simulink model "case7"  (R2024b)
settings: Solver=FixedStepAuto  StartTime=0  StopTime=1  FixedStep=1e-7  RelTol=1e-3
values from neighbouring files (symbols this model uses):
  SG_D_1_D = 0.01056    [IEEE9_case_parameters.m]    (also in case1_parameters.m; case2_parameters.m; case3_parameters.m; case4_parameters.m)
  SG_D_1_EnableSaturation = 0    [IEEE9_case_parameters.m]    (also in case1_parameters.m; case2_parameters.m; case3_parameters.m; case4_parameters.m)
  SG_D_1_f0 = 60    [IEEE9_case_parameters.m]    (also in case1_parameters.m; case2_parameters.m; case3_parameters.m; case4_parameters.m)
  SG_D_1_H = 7.5    [IEEE9_case_parameters.m]    (also in case1_parameters.m; case2_parameters.m; case3_parameters.m; case4_parameters.m)
  SG_D_1_K_A = 20    [IEEE9_case_parameters.m]    (also in case1_parameters.m; case2_parameters.m; case3_parameters.m; case4_parameters.m)
  SG_D_1_K_E = 1.000000e+1    (= 10)    [IEEE9_case_parameters.m]    (also in case1_parameters.m; case2_parameters.m; case3_parameters.m; case4_parameters.m)
  SG_D_1_K_F = 2.363    [IEEE9_case_parameters.m]    (also in case1_parameters.m; case2_parameters.m; case3_parameters.m; case4_parameters.m)
  SG_D_1_K_s = 0.5    [IEEE9_case_parameters.m]    (also in case1_parameters.m = 5; case2_parameters.m = 5; case3_parameters.m = 5; case4_parameters.m = 5)
  SG_D_1_R_a = 0.001088    [IEEE9_case_parameters.m]    (also in case1_parameters.m; case2_parameters.m; case3_parameters.m; case4_parameters.m)
  SG_D_1_S_A = 1    [IEEE9_case_parameters.m]    (also in case1_parameters.m; case2_parameters.m; case3_parameters.m; case4_parameters.m)
  SG_D_1_S_B = 0.103    [IEEE9_case_parameters.m]    (also in case1_parameters.m; case2_parameters.m; case3_parameters.m; case4_parameters.m)
  SG_D_1_S_N = 10.659857    [IEEE9_case_parameters.m]    (also in case1_parameters.m; case2_parameters.m; case3_parameters.m; case4_parameters.m)
  SG_D_1_SpeedPara = 200    [IEEE9_case_parameters.m]    (also in case1_parameters.m; case2_parameters.m; case3_parameters.m; case4_parameters.m)
  SG_D_1_T_0 = 0.720173    [IEEE9_case_parameters.m]    (also in case1_parameters.m = 0.755522; case2_parameters.m = 0.808931; case3_parameters.m = 0.869402; case4_parameters.m = 0.729316)
  SG_D_1_T_1 = 0.3    [IEEE9_case_parameters.m]    (also in case1_parameters.m; case2_parameters.m; case3_parameters.m; case4_parameters.m)
  SG_D_1_T_2 = 0.05    [IEEE9_case_parameters.m]    (also in case1_parameters.m; case2_parameters.m; case3_parameters.m; case4_parameters.m)
  SG_D_1_T_3 = 0.02    [IEEE9_case_parameters.m]    (also in case1_parameters.m; case2_parameters.m; case3_parameters.m; case4_parameters.m)
  SG_D_1_T_4 = 0.005    [IEEE9_case_parameters.m]    (also in case1_parameters.m; case2_parameters.m; case3_parameters.m; case4_parameters.m)
  SG_D_1_T_A = 0.02    [IEEE9_case_parameters.m]    (also in case1_parameters.m; case2_parameters.m; case3_parameters.m; case4_parameters.m)
  SG_D_1_T_dd = 8.000000e+0    (= 8)    [IEEE9_case_parameters.m]    (also in case1_parameters.m; case2_parameters.m; case3_parameters.m; case4_parameters.m)
  SG_D_1_T_ddd = 0.04    [IEEE9_case_parameters.m]    (also in case1_parameters.m; case2_parameters.m; case3_parameters.m; case4_parameters.m)
  SG_D_1_T_E = 0.314    [IEEE9_case_parameters.m]    (also in case1_parameters.m; case2_parameters.m; case3_parameters.m; case4_parameters.m)
  SG_D_1_T_F = 0.35    [IEEE9_case_parameters.m]    (also in case1_parameters.m; case2_parameters.m; case3_parameters.m; case4_parameters.m)
  SG_D_1_T_qd = 0.8    [IEEE9_case_parameters.m]    (also in case1_parameters.m; case2_parameters.m; case3_parameters.m; case4_parameters.m)
  SG_D_1_T_qdd = 0.02    [IEEE9_case_parameters.m]    (also in case1_parameters.m; case2_parameters.m; case3_parameters.m; case4_parameters.m)
  SG_D_1_T_speed = 0.1    [IEEE9_case_parameters.m]    (also in case1_parameters.m = 200; case2_parameters.m = 200; case3_parameters.m = 200; case4_parameters.m = 200)
  SG_D_1_T_w = 0.5    [IEEE9_case_parameters.m]    (also in case1_parameters.m; case2_parameters.m; case3_parameters.m; case4_parameters.m)
  SG_D_1_V_ref = 1.990276    [IEEE9_case_parameters.m]    (also in case1_parameters.m = 2.042296; case2_parameters.m = 2.051388; case3_parameters.m = 2.089584; case4_parameters.m = 2.01845)
  SG_D_1_w_ref = 376.991118    [IEEE9_case_parameters.m]    (also in case1_parameters.m; case2_parameters.m; case3_parameters.m; case4_parameters.m)
  SG_D_1_wb = 6.000000e+1    (= 60)    [IEEE9_case_parameters.m]    (also in case1_parameters.m; case2_parameters.m; case3_parameters.m; case4_parameters.m)
  SG_D_1_x_d = 1.9    [IEEE9_case_parameters.m]    (also in case1_parameters.m; case2_parameters.m; case3_parameters.m; case4_parameters.m)
  SG_D_1_x_dd = 0.302    [IEEE9_case_parameters.m]    (also in case1_parameters.m; case2_parameters.m; case3_parameters.m; case4_parameters.m)
  SG_D_1_x_ddd = 0.204    [IEEE9_case_parameters.m]    (also in case1_parameters.m; case2_parameters.m; case3_parameters.m; case4_parameters.m)
  SG_D_1_x_l = 0.05    [IEEE9_case_parameters.m]    (also in case1_parameters.m; case2_parameters.m; case3_parameters.m; case4_parameters.m)
  SG_D_1_x_q = 1.3    [IEEE9_case_parameters.m]    (also in case1_parameters.m; case2_parameters.m; case3_parameters.m; case4_parameters.m)
  SG_D_1_x_qd = 0.5    [IEEE9_case_parameters.m]    (also in case1_parameters.m; case2_parameters.m; case3_parameters.m; case4_parameters.m)
  SG_D_1_x_qdd = 0.3    [IEEE9_case_parameters.m]    (also in case1_parameters.m; case2_parameters.m; case3_parameters.m; case4_parameters.m)
  SG_D_2_D = 0.02    [IEEE9_case_parameters.m]    (also in case1_parameters.m; case2_parameters.m; case3_parameters.m; case4_parameters.m)
  SG_D_2_EnableSaturation = 0    [IEEE9_case_parameters.m]    (also in case1_parameters.m; case2_parameters.m; case3_parameters.m; case4_parameters.m)
  SG_D_2_f0 = 60    [IEEE9_case_parameters.m]    (also in case1_parameters.m; case2_parameters.m; case3_parameters.m; case4_parameters.m)
  SG_D_2_H = 8.000000e+0    (= 8)    [IEEE9_case_parameters.m]    (also in case1_parameters.m; case2_parameters.m; case3_parameters.m; case4_parameters.m)
  SG_D_2_K_A = 20    [IEEE9_case_parameters.m]    (also in case1_parameters.m; case2_parameters.m; case3_parameters.m; case4_parameters.m)
  SG_D_2_K_E = 1.000000e+1    (= 10)    [IEEE9_case_parameters.m]    (also in case1_parameters.m; case2_parameters.m; case3_parameters.m; case4_parameters.m)
  SG_D_2_K_F = 2.363    [IEEE9_case_parameters.m]    (also in case1_parameters.m; case2_parameters.m; case3_parameters.m; case4_parameters.m)
  SG_D_2_K_s = 0.5    [IEEE9_case_parameters.m]    (also in case1_parameters.m = 4; case2_parameters.m = 4; case3_parameters.m = 4; case4_parameters.m = 4)
  SG_D_2_R_a = 0.001088    [IEEE9_case_parameters.m]    (also in case1_parameters.m; case2_parameters.m; case3_parameters.m; case4_parameters.m)
  SG_D_2_S_A = 1    [IEEE9_case_parameters.m]    (also in case1_parameters.m; case2_parameters.m; case3_parameters.m; case4_parameters.m)
  SG_D_2_S_B = 0.103    [IEEE9_case_parameters.m]    (also in case1_parameters.m; case2_parameters.m; case3_parameters.m; case4_parameters.m)
  SG_D_2_S_N = 10.659857    [IEEE9_case_parameters.m]    (also in case1_parameters.m; case2_parameters.m; case3_parameters.m; case4_parameters.m)
  SG_D_2_SpeedPara = 200    [IEEE9_case_parameters.m]    (also in case1_parameters.m; case2_parameters.m; case3_parameters.m; case4_parameters.m)
  SG_D_2_T_0 = 1.632913    [IEEE9_case_parameters.m]    (also in case1_parameters.m = 1.632925; case2_parameters.m = 1.632915; case3_parameters.m = 1.632914; case4_parameters.m = 1.632927)
  SG_D_2_T_1 = 0.2    [IEEE9_case_parameters.m]    (also in case1_parameters.m; case2_parameters.m; case3_parameters.m; case4_parameters.m)
  SG_D_2_T_2 = 0.05    [IEEE9_case_parameters.m]    (also in case1_parameters.m; case2_parameters.m; case3_parameters.m; case4_parameters.m)
  SG_D_2_T_3 = 0.02    [IEEE9_case_parameters.m]    (also in case1_parameters.m; case2_parameters.m; case3_parameters.m; case4_parameters.m)
  SG_D_2_T_4 = 0.005    [IEEE9_case_parameters.m]    (also in case1_parameters.m; case2_parameters.m; case3_parameters.m; case4_parameters.m)
  SG_D_2_T_A = 0.02    [IEEE9_case_parameters.m]    (also in case1_parameters.m; case2_parameters.m; case3_parameters.m; case4_parameters.m)
  SG_D_2_T_dd = 7.9    [IEEE9_case_parameters.m]    (also in case1_parameters.m; case2_parameters.m; case3_parameters.m; case4_parameters.m)
  SG_D_2_T_ddd = 0.04    [IEEE9_case_parameters.m]    (also in case1_parameters.m; case2_parameters.m; case3_parameters.m; case4_parameters.m)
  SG_D_2_T_E = 0.314    [IEEE9_case_parameters.m]    (also in case1_parameters.m; case2_parameters.m; case3_parameters.m; case4_parameters.m)
  SG_D_2_T_F = 0.35    [IEEE9_case_parameters.m]    (also in case1_parameters.m; case2_parameters.m; case3_parameters.m; case4_parameters.m)
  SG_D_2_T_qd = 0.8    [IEEE9_case_parameters.m]    (also in case1_parameters.m; case2_parameters.m; case3_parameters.m; case4_parameters.m)
  SG_D_2_T_qdd = 0.015    [IEEE9_case_parameters.m]    (also in case1_parameters.m; case2_parameters.m; case3_parameters.m; case4_parameters.m)
  SG_D_2_T_speed = 0.1    [IEEE9_case_parameters.m]    (also in case1_parameters.m = 150; case2_parameters.m = 150; case3_parameters.m = 150; case4_parameters.m = 150)
  SG_D_2_T_w = 0.35    [IEEE9_case_parameters.m]    (also in case1_parameters.m; case2_parameters.m; case3_parameters.m; case4_parameters.m)
  SG_D_2_V_ref = 2.58547    [IEEE9_case_parameters.m]    (also in case1_parameters.m = 2.597896; case2_parameters.m = 2.587136; case3_parameters.m = 2.586042; case4_parameters.m = 2.599679)
  SG_D_2_w_ref = 376.991118    [IEEE9_case_parameters.m]    (also in case1_parameters.m; case2_parameters.m; case3_parameters.m; case4_parameters.m)
  SG_D_2_wb = 6.000000e+1    (= 60)    [IEEE9_case_parameters.m]    (also in case1_parameters.m; case2_parameters.m; case3_parameters.m; case4_parameters.m)
  SG_D_2_x_d = 1.8    [IEEE9_case_parameters.m]    (also in case1_parameters.m; case2_parameters.m; case3_parameters.m; case4_parameters.m)
  SG_D_2_x_dd = 0.302    [IEEE9_case_parameters.m]    (also in case1_parameters.m; case2_parameters.m; case3_parameters.m; case4_parameters.m)
  SG_D_2_x_ddd = 0.204    [IEEE9_case_parameters.m]    (also in case1_parameters.m; case2_parameters.m; case3_parameters.m; case4_parameters.m)
  SG_D_2_x_l = 0.05    [IEEE9_case_parameters.m]    (also in case1_parameters.m; case2_parameters.m; case3_parameters.m; case4_parameters.m)
  SG_D_2_x_q = 1.25    [IEEE9_case_parameters.m]    (also in case1_parameters.m; case2_parameters.m; case3_parameters.m; case4_parameters.m)
  SG_D_2_x_qd = 0.5    [IEEE9_case_parameters.m]    (also in case1_parameters.m; case2_parameters.m; case3_parameters.m; case4_parameters.m)
  SG_D_2_x_qdd = 0.3    [IEEE9_case_parameters.m]    (also in case1_parameters.m; case2_parameters.m; case3_parameters.m; case4_parameters.m)
  SG_D_3_D = 0.02    [IEEE9_case_parameters.m]    (also in case1_parameters.m; case2_parameters.m; case3_parameters.m; case4_parameters.m)
  SG_D_3_EnableSaturation = 0    [IEEE9_case_parameters.m]    (also in case1_parameters.m; case2_parameters.m; case3_parameters.m; case4_parameters.m)
  SG_D_3_f0 = 60    [IEEE9_case_parameters.m]    (also in case1_parameters.m; case2_parameters.m; case3_parameters.m; case4_parameters.m)
  SG_D_3_H = 7.7    [IEEE9_case_parameters.m]    (also in case1_parameters.m; case2_parameters.m; case3_parameters.m; case4_parameters.m)
  SG_D_3_K_A = 20    [IEEE9_case_parameters.m]    (also in case1_parameters.m; case2_parameters.m; case3_parameters.m; case4_parameters.m)
  SG_D_3_K_E = 1.000000e+1    (= 10)    [IEEE9_case_parameters.m]    (also in case1_parameters.m; case2_parameters.m; case3_parameters.m; case4_parameters.m)
  SG_D_3_K_F = 2.363    [IEEE9_case_parameters.m]    (also in case1_parameters.m; case2_parameters.m; case3_parameters.m; case4_parameters.m)
  SG_D_3_K_s = 0.2    [IEEE9_case_parameters.m]    (also in case1_parameters.m = 2; case2_parameters.m = 2; case3_parameters.m = 2; case4_parameters.m = 2)
  SG_D_3_R_a = 0.001088    [IEEE9_case_parameters.m]    (also in case1_parameters.m; case2_parameters.m; case3_parameters.m; case4_parameters.m)
  SG_D_3_S_A = 1    [IEEE9_case_parameters.m]    (also in case1_parameters.m; case2_parameters.m; case3_parameters.m; case4_parameters.m)
  SG_D_3_S_B = 0.103    [IEEE9_case_parameters.m]    (also in case1_parameters.m; case2_parameters.m; case3_parameters.m; case4_parameters.m)
  SG_D_3_S_N = 10.659857    [IEEE9_case_parameters.m]    (also in case1_parameters.m; case2_parameters.m; case3_parameters.m; case4_parameters.m)
  SG_D_3_SpeedPara = 200    [IEEE9_case_parameters.m]    (also in case1_parameters.m; case2_parameters.m; case3_parameters.m; case4_parameters.m)
  SG_D_3_T_0 = 0.850788    [IEEE9_case_parameters.m]    (also in case1_parameters.m = 0.850786; case2_parameters.m = 0.850787; case3_parameters.m; case4_parameters.m = 0.850786)
  SG_D_3_T_1 = 0.2    [IEEE9_case_parameters.m]    (also in case1_parameters.m; case2_parameters.m; case3_parameters.m; case4_parameters.m)
  SG_D_3_T_2 = 0.05    [IEEE9_case_parameters.m]    (also in case1_parameters.m; case2_parameters.m; case3_parameters.m; case4_parameters.m)
  SG_D_3_T_3 = 0.02    [IEEE9_case_parameters.m]    (also in case1_parameters.m; case2_parameters.m; case3_parameters.m; case4_parameters.m)
  SG_D_3_T_4 = 0.005    [IEEE9_case_parameters.m]    (also in case1_parameters.m; case2_parameters.m; case3_parameters.m; case4_parameters.m)
  SG_D_3_T_A = 0.02    [IEEE9_case_parameters.m]    (also in case1_parameters.m; case2_parameters.m; case3_parameters.m; case4_parameters.m)
  SG_D_3_T_dd = 8.1    [IEEE9_case_parameters.m]    (also in case1_parameters.m; case2_parameters.m; case3_parameters.m; case4_parameters.m)
  SG_D_3_T_ddd = 0.04    [IEEE9_case_parameters.m]    (also in case1_parameters.m; case2_parameters.m; case3_parameters.m; case4_parameters.m)
  SG_D_3_T_E = 0.314    [IEEE9_case_parameters.m]    (also in case1_parameters.m; case2_parameters.m; case3_parameters.m; case4_parameters.m)
  SG_D_3_T_F = 0.35    [IEEE9_case_parameters.m]    (also in case1_parameters.m; case2_parameters.m; case3_parameters.m; case4_parameters.m)
  SG_D_3_T_qd = 0.8    [IEEE9_case_parameters.m]    (also in case1_parameters.m; case2_parameters.m; case3_parameters.m; case4_parameters.m)
  SG_D_3_T_qdd = 0.015    [IEEE9_case_parameters.m]    (also in case1_parameters.m; case2_parameters.m; case3_parameters.m; case4_parameters.m)
  SG_D_3_T_speed = 0.1    [IEEE9_case_parameters.m]    (also in case1_parameters.m = 180; case2_parameters.m = 180; case3_parameters.m = 180; case4_parameters.m = 180)
  SG_D_3_T_w = 0.4    [IEEE9_case_parameters.m]    (also in case1_parameters.m; case2_parameters.m; case3_parameters.m; case4_parameters.m)
  SG_D_3_V_ref = 1.892727    [IEEE9_case_parameters.m]    (also in case1_parameters.m = 1.906439; case2_parameters.m = 1.895535; case3_parameters.m = 1.892105; case4_parameters.m = 1.906598)
  SG_D_3_w_ref = 376.991118    [IEEE9_case_parameters.m]    (also in case1_parameters.m; case2_parameters.m; case3_parameters.m; case4_parameters.m)
  SG_D_3_wb = 6.000000e+1    (= 60)    [IEEE9_case_parameters.m]    (also in case1_parameters.m; case2_parameters.m; case3_parameters.m; case4_parameters.m)
  SG_D_3_x_d = 1.85    [IEEE9_case_parameters.m]    (also in case1_parameters.m; case2_parameters.m; case3_parameters.m; case4_parameters.m)
  SG_D_3_x_dd = 0.302    [IEEE9_case_parameters.m]    (also in case1_parameters.m; case2_parameters.m; case3_parameters.m; case4_parameters.m)
  SG_D_3_x_ddd = 0.204    [IEEE9_case_parameters.m]    (also in case1_parameters.m; case2_parameters.m; case3_parameters.m; case4_parameters.m)
  SG_D_3_x_l = 0.05    [IEEE9_case_parameters.m]    (also in case1_parameters.m; case2_parameters.m; case3_parameters.m; case4_parameters.m)
  SG_D_3_x_q = 1.2    [IEEE9_case_parameters.m]    (also in case1_parameters.m; case2_parameters.m; case3_parameters.m; case4_parameters.m)
  SG_D_3_x_qd = 0.5    [IEEE9_case_parameters.m]    (also in case1_parameters.m; case2_parameters.m; case3_parameters.m; case4_parameters.m)
  SG_D_3_x_qdd = 0.3    [IEEE9_case_parameters.m]    (also in case1_parameters.m; case2_parameters.m; case3_parameters.m; case4_parameters.m)
(part 3 of 12)

== system case7/AC_1/d_id_load_7_block ==
  note: d_id_load_7 in case7
      | $376.991118430775\,\mathrm{iq}_{\mathrm{load},7}-1183.31185407349\,\mathrm{id}_{\mathrm{load},7}+1325.75163865199\,\mathrm{vd}_{\mathrm{bus},7}$
      | Automatically generated on 2025-10-31 19:27:23 .
  State_id_load_7_f12d4 : Inport
  State_iq_load_7_dd7e6 : Inport  Port=2
  State_vd_bus_7_f2578 : Inport  Port=3
  Add_9644d : Sum
  Add_dc3b8 : Sum
  Constant_-1183.31185407349_df6cb : Constant  Value=-1183.31185407349
  Constant_1325.75163865199_2375e : Constant  Value=1325.75163865199
  Constant_376.991118430775_db960 : Constant  Value=376.991118430775
  Product_51e76 : Product
  Product_6f4c5 : Product
  Product_99a20 : Product
  Blockout_d_id_load_7_72daa : Outport
  wires:
  Constant_-1183.31185407349_df6cb/1 -> Product_6f4c5/1
  Product_99a20/1 -> Add_dc3b8/2
  State_id_load_7_f12d4/1 -> Product_6f4c5/2
  Constant_376.991118430775_db960/1 -> Product_99a20/1
  Product_6f4c5/1 -> Add_dc3b8/1
  State_iq_load_7_dd7e6/1 -> Product_99a20/2
  Constant_1325.75163865199_2375e/1 -> Product_51e76/1
  State_vd_bus_7_f2578/1 -> Product_51e76/2
  Add_dc3b8/1 -> Add_9644d/1
  Product_51e76/1 -> Add_9644d/2
  Add_9644d/1 -> Blockout_d_id_load_7_72daa/1

== system case7/AC_1/d_id_load_9_block ==
  note: d_id_load_9 in case7
      | $376.991118430775\,\mathrm{iq}_{\mathrm{load},9}-1035.39787233511\,\mathrm{id}_{\mathrm{load},9}+1571.97013638063\,\mathrm{vd}_{\mathrm{bus},9}$
      | Automatically generated on 2025-10-31 19:27:27 .
  State_id_load_9_96eb2 : Inport
  State_iq_load_9_6adcd : Inport  Port=2
  State_vd_bus_9_88276 : Inport  Port=3
  Add_00e07 : Sum
  Add_2d69c : Sum
  Constant_-1035.39787233511_99b41 : Constant  Value=-1035.39787233511
  Constant_1571.97013638063_2807c : Constant  Value=1571.97013638063
  Constant_376.991118430775_e3720 : Constant  Value=376.991118430775
  Product_67593 : Product
  Product_89b93 : Product
  Product_a656a : Product
  Blockout_d_id_load_9_904a9 : Outport
  wires:
  Constant_-1035.39787233511_99b41/1 -> Product_67593/1
  Product_89b93/1 -> Add_00e07/2
  State_id_load_9_96eb2/1 -> Product_67593/2
  Constant_376.991118430775_e3720/1 -> Product_89b93/1
  Product_67593/1 -> Add_00e07/1
  State_iq_load_9_6adcd/1 -> Product_89b93/2
  Constant_1571.97013638063_2807c/1 -> Product_a656a/1
  State_vd_bus_9_88276/1 -> Product_a656a/2
  Add_00e07/1 -> Add_2d69c/1
  Product_a656a/1 -> Add_2d69c/2
  Add_2d69c/1 -> Blockout_d_id_load_9_904a9/1

== system case7/AC_1/d_iq_line_1_4_block ==
  note: d_iq_line_1_4 in case7
      | $6520.85548321271\,\mathrm{vq}_{\mathrm{bus},1}-376.991118430775\,\mathrm{id}_{\mathrm{line},1,4}-6520.85548321271\,\mathrm{vq}_{\mathrm{bus},4}$
      | Automatically generated on 2025-10-31 19:27:32 .
  State_id_line_1_4_2037f : Inport
  State_vq_bus_1_e30e3 : Inport  Port=2
  State_vq_bus_4_e9fbb : Inport  Port=3
  Add_b293c : Sum
  Constant_-376.991118430775_008f9 : Constant  Value=-376.991118430775
  Constant_6520.85548321271_751a6 : Constant  Value=6520.85548321271
  Constant_6520.85548321271_d14b9 : Constant  Value=6520.85548321271
  Product_3db56 : Product
  Product_af949 : Product
  Product_d3f3b : Product
  Subtract_258fd : Sum  Inputs=+-
  Blockout_d_iq_line_1_4_21ed7 : Outport
  wires:
  Constant_-376.991118430775_008f9/1 -> Product_af949/1
  Product_3db56/1 -> Add_b293c/2
  State_id_line_1_4_2037f/1 -> Product_af949/2
  Constant_6520.85548321271_d14b9/1 -> Product_3db56/1
  Product_af949/1 -> Add_b293c/1
  Subtract_258fd/1 -> Blockout_d_iq_line_1_4_21ed7/1
  State_vq_bus_1_e30e3/1 -> Product_3db56/2
  Constant_6520.85548321271_751a6/1 -> Product_d3f3b/1
  State_vq_bus_4_e9fbb/1 -> Product_d3f3b/2
  Add_b293c/1 -> Subtract_258fd/1
  Product_d3f3b/1 -> Subtract_258fd/2

== system case7/AC_1/d_iq_line_3_6_block ==
  note: d_iq_line_3_6 in case7
      | $6409.57808588826\,\mathrm{vq}_{\mathrm{bus},3}-376.991118430775\,\mathrm{id}_{\mathrm{line},3,6}-6409.57808588826\,\mathrm{vq}_{\mathrm{bus},6}$
      | Automatically generated on 2025-10-31 19:27:42 .
  State_id_line_3_6_67359 : Inport
  State_vq_bus_3_71d2c : Inport  Port=2
  State_vq_bus_6_fdbe6 : Inport  Port=3
  Add_a0022 : Sum
  Constant_-376.991118430775_ae57f : Constant  Value=-376.991118430775
  Constant_6409.57808588826_0f654 : Constant  Value=6409.57808588826
  Constant_6409.57808588826_46afb : Constant  Value=6409.57808588826
  Product_1825c : Product
  Product_200c8 : Product
  Product_d047b : Product
  Subtract_9ffe6 : Sum  Inputs=+-
  Blockout_d_iq_line_3_6_d1d92 : Outport
  wires:
  Constant_-376.991118430775_ae57f/1 -> Product_200c8/1
  Product_d047b/1 -> Add_a0022/2
  State_id_line_3_6_67359/1 -> Product_200c8/2
  Constant_6409.57808588826_46afb/1 -> Product_d047b/1
  Product_200c8/1 -> Add_a0022/1
  State_vq_bus_3_71d2c/1 -> Product_d047b/2
  Constant_6409.57808588826_0f654/1 -> Product_1825c/1
  State_vq_bus_6_fdbe6/1 -> Product_1825c/2
  Add_a0022/1 -> Subtract_9ffe6/1
  Product_1825c/1 -> Subtract_9ffe6/2
  Subtract_9ffe6/1 -> Blockout_d_iq_line_3_6_d1d92/1

== system case7/AC_1/d_iq_line_4_5_block ==
  note: d_iq_line_4_5 in case7
      | $4082.62256340274\,\mathrm{vq}_{\mathrm{bus},4}-68.4144322264777\,\mathrm{iq}_{\mathrm{line},4,5}-376.991118430775\,\mathrm{id}_{\mathrm{line},4,5}-4082.62256340274\,\mathrm{vq}_{\mathrm{bus},5}$
      | Automatically generated on 2025-10-31 19:27:35 .
  State_id_line_4_5_fca51 : Inport
  State_iq_line_4_5_74164 : Inport  Port=2
  State_vq_bus_4_9a579 : Inport  Port=3
  State_vq_bus_5_c17cf : Inport  Port=4
  Add_a9a54 : Sum
  Constant_-376.991118430775_541fa : Constant  Value=-376.991118430775
  Constant_4082.62256340274_9a987 : Constant  Value=4082.62256340274
  Constant_4082.62256340274_db37c : Constant  Value=4082.62256340274
  Constant_68.4144322264777_64688 : Constant  Value=68.4144322264777
  Product_0226d : Product
  Product_131fe : Product
  Product_5102d : Product
  Product_581d6 : Product
  Subtract_5bfab : Sum  Inputs=+-
  Subtract_d5959 : Sum  Inputs=+-
  Blockout_d_iq_line_4_5_f0b45 : Outport
  wires:
  Constant_-376.991118430775_541fa/1 -> Product_5102d/1
  Constant_68.4144322264777_64688/1 -> Product_131fe/1
  State_id_line_4_5_fca51/1 -> Product_5102d/2
  State_iq_line_4_5_74164/1 -> Product_131fe/2
  Product_5102d/1 -> Subtract_d5959/1
  Constant_4082.62256340274_9a987/1 -> Product_581d6/1
  Product_131fe/1 -> Subtract_d5959/2
  State_vq_bus_4_9a579/1 -> Product_581d6/2
  Subtract_d5959/1 -> Add_a9a54/1
  Product_581d6/1 -> Add_a9a54/2
  Constant_4082.62256340274_db37c/1 -> Product_0226d/1
  State_vq_bus_5_c17cf/1 -> Product_0226d/2
  Add_a9a54/1 -> Subtract_5bfab/1
  Product_0226d/1 -> Subtract_5bfab/2
  Subtract_5bfab/1 -> Blockout_d_iq_line_4_5_f0b45/1

== system case7/AC_1/d_iq_line_5_6_block ==
  note: d_iq_line_5_6 in case7
      | $2209.41926960619\,\mathrm{vq}_{\mathrm{bus},5}-84.9380563420768\,\mathrm{iq}_{\mathrm{line},5,6}-376.991118430775\,\mathrm{id}_{\mathrm{line},5,6}-2209.41926960619\,\mathrm{vq}_{\mathrm{bus},6}$
      | Automatically generated on 2025-10-31 19:27:39 .
  State_id_line_5_6_a603b : Inport
  State_iq_line_5_6_83796 : Inport  Port=2
  State_vq_bus_5_06daf : Inport  Port=3
  State_vq_bus_6_cbe8b : Inport  Port=4
  Add_9cbe8 : Sum
  Constant_-376.991118430775_c006a : Constant  Value=-376.991118430775
  Constant_2209.41926960619_a5936 : Constant  Value=2209.41926960619
  Constant_2209.41926960619_d0f31 : Constant  Value=2209.41926960619
  Constant_84.9380563420768_bb069 : Constant  Value=84.9380563420768
  Product_08db4 : Product
  Product_850d1 : Product
  Product_9167f : Product
  Product_a68e2 : Product
  Subtract_1d376 : Sum  Inputs=+-
  Subtract_83429 : Sum  Inputs=+-
  Blockout_d_iq_line_5_6_b9d91 : Outport
  wires:
  Constant_-376.991118430775_c006a/1 -> Product_850d1/1
  Constant_84.9380563420768_bb069/1 -> Product_9167f/1
  Subtract_1d376/1 -> Blockout_d_iq_line_5_6_b9d91/1
  State_id_line_5_6_a603b/1 -> Product_850d1/2
  State_iq_line_5_6_83796/1 -> Product_9167f/2
  Product_850d1/1 -> Subtract_83429/1
  Constant_2209.41926960619_a5936/1 -> Product_a68e2/1
  Product_9167f/1 -> Subtract_83429/2
  Product_08db4/1 -> Subtract_1d376/2
  State_vq_bus_5_06daf/1 -> Product_a68e2/2
  Subtract_83429/1 -> Add_9cbe8/1
  Product_a68e2/1 -> Add_9cbe8/2
  Constant_2209.41926960619_d0f31/1 -> Product_08db4/1
  State_vq_bus_6_cbe8b/1 -> Product_08db4/2
  Add_9cbe8/1 -> Subtract_1d376/1

== system case7/AC_1/d_iq_line_6_7_block ==
  note: d_iq_line_6_7 in case7
      | $3726.2031332644\,\mathrm{vq}_{\mathrm{bus},6}-43.7092205891385\,\mathrm{iq}_{\mathrm{line},6,7}-376.991118430775\,\mathrm{id}_{\mathrm{line},6,7}-3726.2031332644\,\mathrm{vq}_{\mathrm{bus},7}$
      | Automatically generated on 2025-10-31 19:27:46 .
  State_id_line_6_7_f0a87 : Inport
  State_iq_line_6_7_8e035 : Inport  Port=2
  State_vq_bus_6_ef30c : Inport  Port=3
  State_vq_bus_7_83713 : Inport  Port=4
  Add_f6c88 : Sum
  Constant_-376.991118430775_931c0 : Constant  Value=-376.991118430775
  Constant_3726.2031332644_26249 : Constant  Value=3726.2031332644
  Constant_3726.2031332644_93a3f : Constant  Value=3726.2031332644
  Constant_43.7092205891385_884b1 : Constant  Value=43.7092205891385
  Product_1b927 : Product
  Product_2b832 : Product
  Product_3c2fa : Product
  Product_a46c8 : Product
  Subtract_20712 : Sum  Inputs=+-
  Subtract_353a1 : Sum  Inputs=+-
  Blockout_d_iq_line_6_7_534ea : Outport
  wires:
  Constant_-376.991118430775_931c0/1 -> Product_3c2fa/1
  Constant_43.7092205891385_884b1/1 -> Product_2b832/1
  State_id_line_6_7_f0a87/1 -> Product_3c2fa/2
  State_iq_line_6_7_8e035/1 -> Product_2b832/2
  Product_3c2fa/1 -> Subtract_20712/1
  Constant_3726.2031332644_26249/1 -> Product_1b927/1
  Product_2b832/1 -> Subtract_20712/2
  State_vq_bus_6_ef30c/1 -> Product_1b927/2
  Subtract_20712/1 -> Add_f6c88/1
  Product_1b927/1 -> Add_f6c88/2
  Constant_3726.2031332644_93a3f/1 -> Product_a46c8/1
  State_vq_bus_7_83713/1 -> Product_a46c8/2
  Add_f6c88/1 -> Subtract_353a1/1
  Product_a46c8/1 -> Subtract_353a1/2
  Subtract_353a1/1 -> Blockout_d_iq_line_6_7_534ea/1

== system case7/AC_1/d_iq_line_7_8_block ==
  note: d_iq_line_7_8 in case7
      | $5216.68438657017\,\mathrm{vq}_{\mathrm{bus},7}-43.7092205891385\,\mathrm{iq}_{\mathrm{line},7,8}-376.991118430775\,\mathrm{id}_{\mathrm{line},7,8}-5216.68438657017\,\mathrm{vq}_{\mathrm{bus},8}$
      | Automatically generated on 2025-10-31 19:27:50 .
  State_id_line_7_8_167a8 : Inport
  State_iq_line_7_8_7ac3b : Inport  Port=2
  State_vq_bus_7_a194e : Inport  Port=3
  State_vq_bus_8_c730a : Inport  Port=4
  Add_7bcb9 : Sum
  Constant_-376.991118430775_8a098 : Constant  Value=-376.991118430775
  Constant_43.7092205891385_492cd : Constant  Value=43.7092205891385
  Constant_5216.68438657017_817d5 : Constant  Value=5216.68438657017
  Constant_5216.68438657017_f2e90 : Constant  Value=5216.68438657017
  Product_1cfac : Product
  Product_454b1 : Product
  Product_6a3ec : Product
  Product_e5fe2 : Product
  Subtract_a467a : Sum  Inputs=+-
  Subtract_e43e1 : Sum  Inputs=+-
  Blockout_d_iq_line_7_8_6dc4f : Outport
  wires:
  Constant_-376.991118430775_8a098/1 -> Product_e5fe2/1
  Constant_43.7092205891385_492cd/1 -> Product_454b1/1
  State_id_line_7_8_167a8/1 -> Product_e5fe2/2
  State_iq_line_7_8_7ac3b/1 -> Product_454b1/2
  Product_e5fe2/1 -> Subtract_a467a/1
  Constant_5216.68438657017_f2e90/1 -> Product_6a3ec/1
  Product_454b1/1 -> Subtract_a467a/2
  State_vq_bus_7_a194e/1 -> Product_6a3ec/2
  Subtract_a467a/1 -> Add_7bcb9/1
  Product_6a3ec/1 -> Add_7bcb9/2
  Constant_5216.68438657017_817d5/1 -> Product_1cfac/1
  State_vq_bus_8_c730a/1 -> Product_1cfac/2
  Add_7bcb9/1 -> Subtract_e43e1/1
  Product_1cfac/1 -> Subtract_e43e1/2
  Subtract_e43e1/1 -> Blockout_d_iq_line_7_8_6dc4f/1

== system case7/AC_1/d_iq_line_8_2_block ==
  note: d_iq_line_8_2 in case7
      | $6009.62041332883\,\mathrm{vq}_{\mathrm{bus},8}-6009.62041332883\,\mathrm{vq}_{\mathrm{bus},2}-376.991118430775\,\mathrm{id}_{\mathrm{line},8,2}$
      | Automatically generated on 2025-10-31 19:27:54 .
  State_id_line_8_2_6be89 : Inport
  State_vq_bus_2_12fee : Inport  Port=2
  State_vq_bus_8_9749c : Inport  Port=3
  Add_ac943 : Sum
  Constant_-376.991118430775_b6a8c : Constant  Value=-376.991118430775
  Constant_6009.62041332883_1bbcb : Constant  Value=6009.62041332883
  Constant_6009.62041332883_43777 : Constant  Value=6009.62041332883
  Product_0162e : Product
  Product_54e83 : Product
  Product_78dd7 : Product
  Subtract_10503 : Sum  Inputs=+-
  Blockout_d_iq_line_8_2_76ae2 : Outport
  wires:
  Constant_-376.991118430775_b6a8c/1 -> Product_54e83/1
  Product_0162e/1 -> Subtract_10503/2
  State_id_line_8_2_6be89/1 -> Product_54e83/2
  Constant_6009.62041332883_43777/1 -> Product_0162e/1
  Product_54e83/1 -> Subtract_10503/1
  State_vq_bus_2_12fee/1 -> Product_0162e/2
  Constant_6009.62041332883_1bbcb/1 -> Product_78dd7/1
  State_vq_bus_8_9749c/1 -> Product_78dd7/2
  Subtract_10503/1 -> Add_ac943/1
  Product_78dd7/1 -> Add_ac943/2
  Add_ac943/1 -> Blockout_d_iq_line_8_2_76ae2/1

== system case7/AC_1/d_iq_line_8_9_block ==
  note: d_iq_line_8_9 in case7
      | $2332.92717908728\,\mathrm{vq}_{\mathrm{bus},8}-73.5886329831021\,\mathrm{iq}_{\mathrm{line},8,9}-376.991118430775\,\mathrm{id}_{\mathrm{line},8,9}-2332.92717908728\,\mathrm{vq}_{\mathrm{bus},9}$
      | Automatically generated on 2025-10-31 19:27:57 .
  State_id_line_8_9_ece40 : Inport
  State_iq_line_8_9_7b378 : Inport  Port=2
  State_vq_bus_8_e5c45 : Inport  Port=3
  State_vq_bus_9_6e5a2 : Inport  Port=4
  Add_c8ccf : Sum
  Constant_-376.991118430775_5848c : Constant  Value=-376.991118430775
  Constant_2332.92717908728_e41d9 : Constant  Value=2332.92717908728
  Constant_2332.92717908728_e4305 : Constant  Value=2332.92717908728
  Constant_73.5886329831021_d2bfe : Constant  Value=73.5886329831021
  Product_0c529 : Product
  Product_5095e : Product
  Product_d4efd : Product
  Product_fd2e5 : Product
  Subtract_0ab39 : Sum  Inputs=+-
  Subtract_80eb0 : Sum  Inputs=+-
  Blockout_d_iq_line_8_9_5ccbd : Outport
  wires:
  Constant_-376.991118430775_5848c/1 -> Product_0c529/1
  Constant_73.5886329831021_d2bfe/1 -> Product_d4efd/1
  State_id_line_8_9_ece40/1 -> Product_0c529/2
  State_iq_line_8_9_7b378/1 -> Product_d4efd/2
  Product_0c529/1 -> Subtract_0ab39/1
  Constant_2332.92717908728_e41d9/1 -> Product_5095e/1
  Product_d4efd/1 -> Subtract_0ab39/2
  State_vq_bus_8_e5c45/1 -> Product_5095e/2
  Subtract_0ab39/1 -> Add_c8ccf/1
  Product_5095e/1 -> Add_c8ccf/2
  Constant_2332.92717908728_e4305/1 -> Product_fd2e5/1
  Add_c8ccf/1 -> Subtract_80eb0/1
  State_vq_bus_9_6e5a2/1 -> Product_fd2e5/2
  Product_fd2e5/1 -> Subtract_80eb0/2
  Subtract_80eb0/1 -> Blockout_d_iq_line_8_9_5ccbd/1

== system case7/AC_1/d_iq_line_9_4_block ==
  note: d_iq_line_9_4 in case7
      | $4418.83853921238\,\mathrm{vq}_{\mathrm{bus},9}-43.5579776113214\,\mathrm{iq}_{\mathrm{line},9,4}-4418.83853921238\,\mathrm{vq}_{\mathrm{bus},4}-376.991118430775\,\mathrm{id}_{\mathrm{line},9,4}$
      | Automatically generated on 2025-10-31 19:28:01 .
  State_id_line_9_4_16341 : Inport
  State_iq_line_9_4_9816b : Inport  Port=2
  State_vq_bus_4_2d516 : Inport  Port=3
  State_vq_bus_9_6157d : Inport  Port=4
  Add_6a82c : Sum
  Constant_-376.991118430775_e8397 : Constant  Value=-376.991118430775
  Constant_43.5579776113214_ec61d : Constant  Value=43.5579776113214
  Constant_4418.83853921238_2d81f : Constant  Value=4418.83853921238
  Constant_4418.83853921238_6a47c : Constant  Value=4418.83853921238
  Product_31185 : Product
  Product_78512 : Product
  Product_865f0 : Product
  Product_cf0f0 : Product
  Subtract_95a16 : Sum  Inputs=+-
  Subtract_b009e : Sum  Inputs=+-
  Blockout_d_iq_line_9_4_4ec5c : Outport
  wires:
  Constant_-376.991118430775_e8397/1 -> Product_cf0f0/1
  Constant_43.5579776113214_ec61d/1 -> Product_78512/1
  State_id_line_9_4_16341/1 -> Product_cf0f0/2
  State_iq_line_9_4_9816b/1 -> Product_78512/2
  Product_cf0f0/1 -> Subtract_95a16/1
  Constant_4418.83853921238_6a47c/1 -> Product_865f0/1
  Product_78512/1 -> Subtract_95a16/2
  State_vq_bus_4_2d516/1 -> Product_865f0/2
  Subtract_95a16/1 -> Subtract_b009e/1
  Product_865f0/1 -> Subtract_b009e/2
  Constant_4418.83853921238_2d81f/1 -> Product_31185/1
  Add_6a82c/1 -> Blockout_d_iq_line_9_4_4ec5c/1
  State_vq_bus_9_6157d/1 -> Product_31185/2
  Subtract_b009e/1 -> Add_6a82c/1
  Product_31185/1 -> Add_6a82c/2

== system case7/AC_1/d_iq_load_5_block ==
  note: d_iq_load_5 in case7
      | $1265.54551301855\,\mathrm{vq}_{\mathrm{bus},5}-1242.47744681877\,\mathrm{iq}_{\mathrm{load},5}-376.991118430775\,\mathrm{id}_{\mathrm{load},5}$
      | Automatically generated on 2025-10-31 19:27:22 .
  State_id_load_5_99883 : Inport
  State_iq_load_5_ceced : Inport  Port=2
  State_vq_bus_5_33ca4 : Inport  Port=3
  Add_46ebe : Sum
  Constant_-376.991118430775_ff2ed : Constant  Value=-376.991118430775
  Constant_1242.47744681877_be5a6 : Constant  Value=1242.47744681877
  Constant_1265.54551301855_d3716 : Constant  Value=1265.54551301855
  Product_07b71 : Product
  Product_5605d : Product
  Product_78a65 : Product
  Subtract_3956b : Sum  Inputs=+-
  Blockout_d_iq_load_5_d6271 : Outport
  wires:
  Constant_-376.991118430775_ff2ed/1 -> Product_07b71/1
  Product_78a65/1 -> Subtract_3956b/2
  State_id_load_5_99883/1 -> Product_07b71/2
  Constant_1242.47744681877_be5a6/1 -> Product_78a65/1
  Product_07b71/1 -> Subtract_3956b/1
  State_iq_load_5_ceced/1 -> Product_78a65/2
  Constant_1265.54551301855_d3716/1 -> Product_5605d/1
  State_vq_bus_5_33ca4/1 -> Product_5605d/2
  Subtract_3956b/1 -> Add_46ebe/1
  Product_5605d/1 -> Add_46ebe/2
  Add_46ebe/1 -> Blockout_d_iq_load_5_d6271/1

== system case7/AC_1/d_iq_load_7_block ==
  note: d_iq_load_7 in case7
      | $1325.75163865199\,\mathrm{vq}_{\mathrm{bus},7}-1183.31185407349\,\mathrm{iq}_{\mathrm{load},7}-376.991118430775\,\mathrm{id}_{\mathrm{load},7}$
      | Automatically generated on 2025-10-31 19:27:25 .
  State_id_load_7_23b97 : Inport
  State_iq_load_7_999fa : Inport  Port=2
  State_vq_bus_7_34020 : Inport  Port=3
  Add_5268c : Sum
  Constant_-376.991118430775_e1af2 : Constant  Value=-376.991118430775
  Constant_1183.31185407349_0009c : Constant  Value=1183.31185407349
  Constant_1325.75163865199_65674 : Constant  Value=1325.75163865199
  Product_441c6 : Product
  Product_4c8d2 : Product
  Product_8f0f0 : Product
  Subtract_8999d : Sum  Inputs=+-
  Blockout_d_iq_load_7_bdd33 : Outport
  wires:
  Constant_-376.991118430775_e1af2/1 -> Product_8f0f0/1
  Product_441c6/1 -> Subtract_8999d/2
  State_id_load_7_23b97/1 -> Product_8f0f0/2
  Constant_1183.31185407349_0009c/1 -> Product_441c6/1
  Product_8f0f0/1 -> Subtract_8999d/1
  State_iq_load_7_999fa/1 -> Product_441c6/2
  Constant_1325.75163865199_65674/1 -> Product_4c8d2/1
  State_vq_bus_7_34020/1 -> Product_4c8d2/2
  Subtract_8999d/1 -> Add_5268c/1
  Product_4c8d2/1 -> Add_5268c/2
  Add_5268c/1 -> Blockout_d_iq_load_7_bdd33/1

== system case7/AC_1/d_iq_load_9_block ==
  note: d_iq_load_9 in case7
      | $1571.97013638063\,\mathrm{vq}_{\mathrm{bus},9}-1035.39787233511\,\mathrm{iq}_{\mathrm{load},9}-376.991118430775\,\mathrm{id}_{\mathrm{load},9}$
      | Automatically generated on 2025-10-31 19:27:28 .
  State_id_load_9_f3e09 : Inport
  State_iq_load_9_40cec : Inport  Port=2
  State_vq_bus_9_28711 : Inport  Port=3
  Add_05624 : Sum
  Constant_-376.991118430775_b6e48 : Constant  Value=-376.991118430775
  Constant_1035.39787233511_471be : Constant  Value=1035.39787233511
  Constant_1571.97013638063_48574 : Constant  Value=1571.97013638063
  Product_0da03 : Product
  Product_21d5b : Product
  Product_9c79b : Product
  Subtract_51327 : Sum  Inputs=+-
  Blockout_d_iq_load_9_4b775 : Outport
  wires:
  Constant_-376.991118430775_b6e48/1 -> Product_0da03/1
  Product_21d5b/1 -> Subtract_51327/2
  State_id_load_9_f3e09/1 -> Product_0da03/2
  Add_05624/1 -> Blockout_d_iq_load_9_4b775/1
  Constant_1035.39787233511_471be/1 -> Product_21d5b/1
  Product_9c79b/1 -> Add_05624/2
  Product_0da03/1 -> Subtract_51327/1
  State_iq_load_9_40cec/1 -> Product_21d5b/2
  Constant_1571.97013638063_48574/1 -> Product_9c79b/1
  State_vq_bus_9_28711/1 -> Product_9c79b/2
  Subtract_51327/1 -> Add_05624/1

== system case7/AC_1/d_vd_bus_1_block ==
  note: d_vd_bus_1 in case7
      | $37699111.8430775\,\mathrm{id}_{\mathrm{bus},1}+376.991118430775\,\mathrm{vq}_{\mathrm{bus},1}$
      | Automatically generated on 2025-10-31 19:26:58 .
  Alge_id_bus_1_aedfe : Inport
  State_vq_bus_1_b64b1 : Inport  Port=2
  Add_a0426 : Sum
  Constant_376.991118430775_a1534 : Constant  Value=376.991118430775
  Constant_37699111.8430775_620b5 : Constant  Value=37699111.8430775
  Product_6370d : Product
  Product_9ad73 : Product
  Blockout_d_vd_bus_1_35ce7 : Outport
  wires:
  Constant_37699111.8430775_620b5/1 -> Product_9ad73/1
  Product_6370d/1 -> Add_a0426/2
  Alge_id_bus_1_aedfe/1 -> Product_9ad73/2
  Constant_376.991118430775_a1534/1 -> Product_6370d/1
  State_vq_bus_1_b64b1/1 -> Product_6370d/2
  Add_a0426/1 -> Blockout_d_vd_bus_1_35ce7/1
  Product_9ad73/1 -> Add_a0426/1

== system case7/AC_1/d_vd_bus_2_block ==
  note: d_vd_bus_2 in case7
      | $37699111.8430775\,\mathrm{id}_{\mathrm{bus},2}+376.991118430775\,\mathrm{vq}_{\mathrm{bus},2}$
      | Automatically generated on 2025-10-31 19:27:00 .
  Alge_id_bus_2_e0197 : Inport
  State_vq_bus_2_07e0b : Inport  Port=2
  Add_a306a : Sum
  Constant_376.991118430775_d4e29 : Constant  Value=376.991118430775
  Constant_37699111.8430775_a775d : Constant  Value=37699111.8430775
  Product_d9b46 : Product
  Product_f18a8 : Product
  Blockout_d_vd_bus_2_06f1a : Outport
  wires:
  Constant_37699111.8430775_a775d/1 -> Product_d9b46/1
  Product_f18a8/1 -> Add_a306a/2
  Alge_id_bus_2_e0197/1 -> Product_d9b46/2
  Constant_376.991118430775_d4e29/1 -> Product_f18a8/1
  Product_d9b46/1 -> Add_a306a/1
  State_vq_bus_2_07e0b/1 -> Product_f18a8/2
  Add_a306a/1 -> Blockout_d_vd_bus_2_06f1a/1

== system case7/AC_1/d_vd_bus_3_block ==
  note: d_vd_bus_3 in case7
      | $37699111.8430775\,\mathrm{id}_{\mathrm{bus},3}+376.991118430775\,\mathrm{vq}_{\mathrm{bus},3}$
      | Automatically generated on 2025-10-31 19:27:03 .
  Alge_id_bus_3_35d15 : Inport
  State_vq_bus_3_28960 : Inport  Port=2
  Add_ddac0 : Sum
  Constant_376.991118430775_e75bd : Constant  Value=376.991118430775
  Constant_37699111.8430775_7dfc8 : Constant  Value=37699111.8430775
  Product_28b4a : Product
  Product_d763c : Product
  Blockout_d_vd_bus_3_2695b : Outport
  wires:
  Constant_37699111.8430775_7dfc8/1 -> Product_28b4a/1
  Product_d763c/1 -> Add_ddac0/2
  Alge_id_bus_3_35d15/1 -> Product_28b4a/2
  Constant_376.991118430775_e75bd/1 -> Product_d763c/1
  Product_28b4a/1 -> Add_ddac0/1
  State_vq_bus_3_28960/1 -> Product_d763c/2
  Add_ddac0/1 -> Blockout_d_vd_bus_3_2695b/1

== system case7/AC_1/d_vd_bus_4_block ==
  note: d_vd_bus_4 in case7
      | $2257.43184689087\,\mathrm{id}_{\mathrm{bus},4}+376.991118430775\,\mathrm{vq}_{\mathrm{bus},4}$
      | Automatically generated on 2025-10-31 19:27:06 .
  Alge_id_bus_4_bf9d1 : Inport
  State_vq_bus_4_a32d2 : Inport  Port=2
  Add_4a57b : Sum
  Constant_2257.43184689087_b5a50 : Constant  Value=2257.43184689087
  Constant_376.991118430775_98cc8 : Constant  Value=376.991118430775
  Product_c40e9 : Product
  Product_e6fb9 : Product
  Blockout_d_vd_bus_4_77c2e : Outport
  wires:
  Constant_2257.43184689087_b5a50/1 -> Product_e6fb9/1
  Product_c40e9/1 -> Add_4a57b/2
  Alge_id_bus_4_bf9d1/1 -> Product_e6fb9/2
  Constant_376.991118430775_98cc8/1 -> Product_c40e9/1
  Product_e6fb9/1 -> Add_4a57b/1
  State_vq_bus_4_a32d2/1 -> Product_c40e9/2
  Add_4a57b/1 -> Blockout_d_vd_bus_4_77c2e/1

== system case7/AC_1/d_vd_bus_5_block ==
  note: d_vd_bus_5 in case7
      | $1461.2058853906\,\mathrm{id}_{\mathrm{bus},5}+376.991118430775\,\mathrm{vq}_{\mathrm{bus},5}$
      | Automatically generated on 2025-10-31 19:27:08 .
  Alge_id_bus_5_39b8d : Inport
  State_vq_bus_5_e58cb : Inport  Port=2
  Add_8655d : Sum
  Constant_1461.2058853906_8ec46 : Constant  Value=1461.2058853906
  Constant_376.991118430775_2ef42 : Constant  Value=376.991118430775
  Product_0d3b7 : Product
  Product_2dc89 : Product
  Blockout_d_vd_bus_5_8bd9d : Outport
  wires:
  Constant_1461.2058853906_8ec46/1 -> Product_2dc89/1
  Product_0d3b7/1 -> Add_8655d/2
  Alge_id_bus_5_39b8d/1 -> Product_2dc89/2
  Constant_376.991118430775_2ef42/1 -> Product_0d3b7/1
  Product_2dc89/1 -> Add_8655d/1
  State_vq_bus_5_e58cb/1 -> Product_0d3b7/2
  Add_8655d/1 -> Blockout_d_vd_bus_5_8bd9d/1

== system case7/AC_1/d_vd_bus_6_block ==
  note: d_vd_bus_6 in case7
      | $1329.77466818616\,\mathrm{id}_{\mathrm{bus},6}+376.991118430775\,\mathrm{vq}_{\mathrm{bus},6}$
      | Automatically generated on 2025-10-31 19:27:10 .
  Alge_id_bus_6_09be4 : Inport
  State_vq_bus_6_b4a62 : Inport  Port=2
  Add_998bb : Sum
  Constant_1329.77466818616_fbd74 : Constant  Value=1329.77466818616
  Constant_376.991118430775_a27f1 : Constant  Value=376.991118430775
  Product_23204 : Product
  Product_2de83 : Product
  Blockout_d_vd_bus_6_17a33 : Outport
  wires:
  Constant_1329.77466818616_fbd74/1 -> Product_2de83/1
  Product_23204/1 -> Add_998bb/2
  Alge_id_bus_6_09be4/1 -> Product_2de83/2
  Constant_376.991118430775_a27f1/1 -> Product_23204/1
  Product_2de83/1 -> Add_998bb/1
  State_vq_bus_6_b4a62/1 -> Product_23204/2
  Add_998bb/1 -> Blockout_d_vd_bus_6_17a33/1

== system case7/AC_1/d_vd_bus_7_block ==
  note: d_vd_bus_7 in case7
      | $2106.09563369148\,\mathrm{id}_{\mathrm{bus},7}+376.991118430775\,\mathrm{vq}_{\mathrm{bus},7}$
      | Automatically generated on 2025-10-31 19:27:13 .
  Alge_id_bus_7_a194e : Inport
  State_vq_bus_7_51f84 : Inport  Port=2
  Add_1012f : Sum
  Constant_2106.09563369148_d5f1f : Constant  Value=2106.09563369148
  Constant_376.991118430775_c1985 : Constant  Value=376.991118430775
  Product_5104c : Product
  Product_d7bad : Product
  Blockout_d_vd_bus_7_db642 : Outport
  wires:
  Constant_2106.09563369148_d5f1f/1 -> Product_5104c/1
  Product_d7bad/1 -> Add_1012f/2
  Alge_id_bus_7_a194e/1 -> Product_5104c/2
  Constant_376.991118430775_c1985/1 -> Product_d7bad/1
  Product_5104c/1 -> Add_1012f/1
  State_vq_bus_7_51f84/1 -> Product_d7bad/2
  Add_1012f/1 -> Blockout_d_vd_bus_7_db642/1

== system case7/AC_1/d_vd_bus_8_block ==
  note: d_vd_bus_8 in case7
      | $1657.10381727813\,\mathrm{id}_{\mathrm{bus},8}+376.991118430775\,\mathrm{vq}_{\mathrm{bus},8}$
      | Automatically generated on 2025-10-31 19:27:15 .
  Alge_id_bus_8_725a0 : Inport
  State_vq_bus_8_d9b83 : Inport  Port=2
  Add_f90e4 : Sum
  Constant_1657.10381727813_86a4d : Constant  Value=1657.10381727813
  Constant_376.991118430775_08379 : Constant  Value=376.991118430775
  Product_4da22 : Product
  Product_5ff5f : Product
  Blockout_d_vd_bus_8_7183e : Outport
  wires:
  Constant_1657.10381727813_86a4d/1 -> Product_4da22/1
  Product_5ff5f/1 -> Add_f90e4/2
  Alge_id_bus_8_725a0/1 -> Product_4da22/2
  Constant_376.991118430775_08379/1 -> Product_5ff5f/1
  Product_4da22/1 -> Add_f90e4/1
  State_vq_bus_8_d9b83/1 -> Product_5ff5f/2
  Add_f90e4/1 -> Blockout_d_vd_bus_8_7183e/1

== system case7/AC_1/d_vd_bus_9_block ==
  note: d_vd_bus_9 in case7
      | $1564.27849971276\,\mathrm{id}_{\mathrm{bus},9}+376.991118430775\,\mathrm{vq}_{\mathrm{bus},9}$
      | Automatically generated on 2025-10-31 19:27:18 .
  Alge_id_bus_9_c43c1 : Inport
  State_vq_bus_9_51ac1 : Inport  Port=2
  Add_68e4f : Sum
  Constant_1564.27849971276_c7fb2 : Constant  Value=1564.27849971276
  Constant_376.991118430775_57dc4 : Constant  Value=376.991118430775
  Product_4f570 : Product
  Product_51272 : Product
  Blockout_d_vd_bus_9_ed3cf : Outport
  wires:
  Constant_1564.27849971276_c7fb2/1 -> Product_51272/1
  Product_4f570/1 -> Add_68e4f/2
  Alge_id_bus_9_c43c1/1 -> Product_51272/2
  Constant_376.991118430775_57dc4/1 -> Product_4f570/1
  Product_51272/1 -> Add_68e4f/1
  State_vq_bus_9_51ac1/1 -> Product_4f570/2
  Add_68e4f/1 -> Blockout_d_vd_bus_9_ed3cf/1

== system case7/AC_1/d_vq_bus_1_block ==
  note: d_vq_bus_1 in case7
      | $37699111.8430775\,\mathrm{iq}_{\mathrm{bus},1}-376.991118430775\,\mathrm{vd}_{\mathrm{bus},1}$
      | Automatically generated on 2025-10-31 19:26:59 .
  Alge_iq_bus_1_697df : Inport
  State_vd_bus_1_3d80d : Inport  Port=2
  Constant_376.991118430775_aecc3 : Constant  Value=376.991118430775
  Constant_37699111.8430775_5ec1d : Constant  Value=37699111.8430775
  Product_14419 : Product
  Product_d8c9a : Product
  Subtract_2f9e6 : Sum  Inputs=+-
  Blockout_d_vq_bus_1_47d83 : Outport
  wires:
  Constant_37699111.8430775_5ec1d/1 -> Product_d8c9a/1
  Constant_376.991118430775_aecc3/1 -> Product_14419/1
  Alge_iq_bus_1_697df/1 -> Product_d8c9a/2
  State_vd_bus_1_3d80d/1 -> Product_14419/2
  Product_d8c9a/1 -> Subtract_2f9e6/1
  Product_14419/1 -> Subtract_2f9e6/2
  Subtract_2f9e6/1 -> Blockout_d_vq_bus_1_47d83/1

== system case7/AC_1/d_vq_bus_2_block ==
  note: d_vq_bus_2 in case7
      | $37699111.8430775\,\mathrm{iq}_{\mathrm{bus},2}-376.991118430775\,\mathrm{vd}_{\mathrm{bus},2}$
      | Automatically generated on 2025-10-31 19:27:02 .
  Alge_iq_bus_2_6bd95 : Inport
  State_vd_bus_2_d11cb : Inport  Port=2
  Constant_376.991118430775_76f8a : Constant  Value=376.991118430775
  Constant_37699111.8430775_af5cd : Constant  Value=37699111.8430775
  Product_77f0b : Product
  Product_c1847 : Product
  Subtract_582b9 : Sum  Inputs=+-
  Blockout_d_vq_bus_2_220e4 : Outport
  wires:
  Constant_37699111.8430775_af5cd/1 -> Product_c1847/1
  Constant_376.991118430775_76f8a/1 -> Product_77f0b/1
  Alge_iq_bus_2_6bd95/1 -> Product_c1847/2
  State_vd_bus_2_d11cb/1 -> Product_77f0b/2
  Product_c1847/1 -> Subtract_582b9/1
  Product_77f0b/1 -> Subtract_582b9/2
  Subtract_582b9/1 -> Blockout_d_vq_bus_2_220e4/1

== system case7/AC_1/d_vq_bus_3_block ==
  note: d_vq_bus_3 in case7
      | $37699111.8430775\,\mathrm{iq}_{\mathrm{bus},3}-376.991118430775\,\mathrm{vd}_{\mathrm{bus},3}$
      | Automatically generated on 2025-10-31 19:27:04 .
  Alge_iq_bus_3_bf354 : Inport
  State_vd_bus_3_03f14 : Inport  Port=2
  Constant_376.991118430775_2cc56 : Constant  Value=376.991118430775
  Constant_37699111.8430775_d73c8 : Constant  Value=37699111.8430775
  Product_30c81 : Product
  Product_b92c1 : Product
  Subtract_d46aa : Sum  Inputs=+-
  Blockout_d_vq_bus_3_782d4 : Outport
  wires:
  Constant_37699111.8430775_d73c8/1 -> Product_b92c1/1
  Constant_376.991118430775_2cc56/1 -> Product_30c81/1
  Alge_iq_bus_3_bf354/1 -> Product_b92c1/2
  State_vd_bus_3_03f14/1 -> Product_30c81/2
  Product_b92c1/1 -> Subtract_d46aa/1
  Product_30c81/1 -> Subtract_d46aa/2
  Subtract_d46aa/1 -> Blockout_d_vq_bus_3_782d4/1

== system case7/AC_1/d_vq_bus_4_block ==
  note: d_vq_bus_4 in case7
      | $2257.43184689087\,\mathrm{iq}_{\mathrm{bus},4}-376.991118430775\,\mathrm{vd}_{\mathrm{bus},4}$
      | Automatically generated on 2025-10-31 19:27:07 .
  Alge_iq_bus_4_08719 : Inport
  State_vd_bus_4_858e6 : Inport  Port=2
  Constant_2257.43184689087_727a2 : Constant  Value=2257.43184689087
  Constant_376.991118430775_d8381 : Constant  Value=376.991118430775
  Product_0bc71 : Product
  Product_35b13 : Product
  Subtract_d35ca : Sum  Inputs=+-
  Blockout_d_vq_bus_4_54be8 : Outport
  wires:
  Constant_2257.43184689087_727a2/1 -> Product_35b13/1
  Constant_376.991118430775_d8381/1 -> Product_0bc71/1
  Alge_iq_bus_4_08719/1 -> Product_35b13/2
  State_vd_bus_4_858e6/1 -> Product_0bc71/2
  Product_35b13/1 -> Subtract_d35ca/1
  Product_0bc71/1 -> Subtract_d35ca/2
  Subtract_d35ca/1 -> Blockout_d_vq_bus_4_54be8/1

== system case7/AC_1/d_vq_bus_5_block ==
  note: d_vq_bus_5 in case7
      | $1461.2058853906\,\mathrm{iq}_{\mathrm{bus},5}-376.991118430775\,\mathrm{vd}_{\mathrm{bus},5}$
      | Automatically generated on 2025-10-31 19:27:09 .
  Alge_iq_bus_5_edb30 : Inport
  State_vd_bus_5_1db70 : Inport  Port=2
  Constant_1461.2058853906_5a0ac : Constant  Value=1461.2058853906
  Constant_376.991118430775_35f9f : Constant  Value=376.991118430775
  Product_0723e : Product
  Product_a8f57 : Product
  Subtract_1bc66 : Sum  Inputs=+-
  Blockout_d_vq_bus_5_ada7d : Outport
  wires:
  Constant_1461.2058853906_5a0ac/1 -> Product_a8f57/1
  Constant_376.991118430775_35f9f/1 -> Product_0723e/1
  Alge_iq_bus_5_edb30/1 -> Product_a8f57/2
  State_vd_bus_5_1db70/1 -> Product_0723e/2
  Product_a8f57/1 -> Subtract_1bc66/1
  Product_0723e/1 -> Subtract_1bc66/2
  Subtract_1bc66/1 -> Blockout_d_vq_bus_5_ada7d/1

== system case7/AC_1/d_vq_bus_6_block ==
  note: d_vq_bus_6 in case7
      | $1329.77466818616\,\mathrm{iq}_{\mathrm{bus},6}-376.991118430775\,\mathrm{vd}_{\mathrm{bus},6}$
      | Automatically generated on 2025-10-31 19:27:11 .
  Alge_iq_bus_6_c1a18 : Inport
  State_vd_bus_6_cf8cd : Inport  Port=2
  Constant_1329.77466818616_f9eb8 : Constant  Value=1329.77466818616
  Constant_376.991118430775_743e9 : Constant  Value=376.991118430775
  Product_0d8d3 : Product
  Product_36895 : Product
  Subtract_8947b : Sum  Inputs=+-
  Blockout_d_vq_bus_6_cdc68 : Outport
  wires:
  Constant_1329.77466818616_f9eb8/1 -> Product_0d8d3/1
  Constant_376.991118430775_743e9/1 -> Product_36895/1
  Alge_iq_bus_6_c1a18/1 -> Product_0d8d3/2
  State_vd_bus_6_cf8cd/1 -> Product_36895/2
  Product_0d8d3/1 -> Subtract_8947b/1
  Product_36895/1 -> Subtract_8947b/2
  Subtract_8947b/1 -> Blockout_d_vq_bus_6_cdc68/1
